simulink model "MLF-VirtualPlatformManualTest"  (R2017b)
settings: Solver=VariableStepAuto  StartTime=0.0  StopTime=inf  RelTol=1e-3
libraries: simulink x3, instrumentlib x2, realtime_pacer_lib x1
settings Model: Creator=twyleg  LastModifiedBy=twyleg

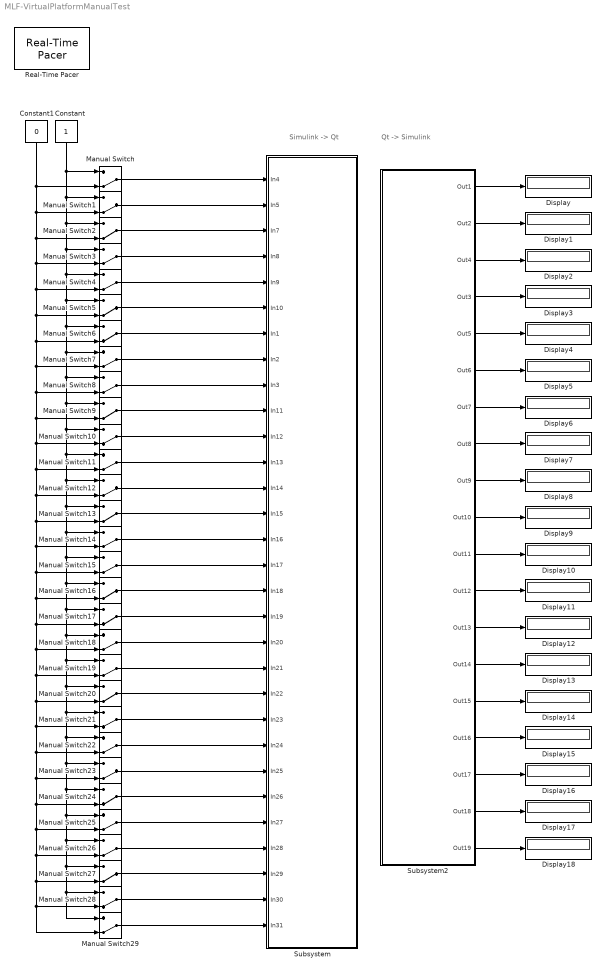
== system MLF-VirtualPlatformManualTest ==
  note: Simulink -> Qt
  note: Qt -> Simulink
  Constant : Constant  OutDataTypeStr=boolean
  Constant1 : Constant  Value=0  OutDataTypeStr=boolean
  Display{,1..18} (19 alike) : Display
  Manual Switch{,1..29} (30 alike) : ManualSwitch  CurrentSetting=0
  Real-Time Pacer : realtime_pacer_lib/Real-Time Pacer  simTimePerRealTime=1
  Subsystem : Subsystem
  Subsystem2 : Subsystem
  wires:
  Subsystem2/1(Out1) -> Display/1
  Subsystem2/2(Out2) -> Display1/1
  Subsystem2/3(Out4) -> Display2/1
  Subsystem2/4(Out3) -> Display3/1
  Subsystem2/5(Out5) -> Display4/1
  Manual Switch/1 -> Subsystem/1(In4)
  Manual Switch1/1 -> Subsystem/2(In5)
  Manual Switch2/1 -> Subsystem/3(In7)
  Manual Switch3/1 -> Subsystem/4(In8)
  Manual Switch4/1 -> Subsystem/5(In9)
  Manual Switch5/1 -> Subsystem/6(In10)
  Manual Switch6/1 -> Subsystem/7(In1)
  Manual Switch7/1 -> Subsystem/8(In2)
  Manual Switch8/1 -> Subsystem/9(In3)
  Manual Switch9/1 -> Subsystem/10(In11)
  Manual Switch10/1 -> Subsystem/11(In12)
  Manual Switch11/1 -> Subsystem/12(In13)
  Manual Switch12/1 -> Subsystem/13(In14)
  Manual Switch13/1 -> Subsystem/14(In15)
  Manual Switch14/1 -> Subsystem/15(In16)
  Manual Switch15/1 -> Subsystem/16(In17)
  Manual Switch16/1 -> Subsystem/17(In18)
  Manual Switch17/1 -> Subsystem/18(In19)
  Manual Switch18/1 -> Subsystem/19(In20)
  Manual Switch19/1 -> Subsystem/20(In21)
  Manual Switch20/1 -> Subsystem/21(In22)
  Manual Switch21/1 -> Subsystem/22(In23)
  Manual Switch22/1 -> Subsystem/23(In24)
  Manual Switch23/1 -> Subsystem/24(In25)
  Manual Switch24/1 -> Subsystem/25(In26)
  Manual Switch25/1 -> Subsystem/26(In27)
  Manual Switch26/1 -> Subsystem/27(In28)
  Manual Switch27/1 -> Subsystem/28(In29)
  Manual Switch28/1 -> Subsystem/29(In30)
  Manual Switch29/1 -> Subsystem/30(In31)
  Constant1/1 -> Manual Switch5/2, Manual Switch6/2, Manual Switch7/2, Manual Switch8/2, Manual Switch9/2, Manual Switch10/2, Manual Switch11/2, Manual Switch12/2, Manual Switch13/2, Manual Switch14/2, Manual Switch15/2, Manual Switch16/2, Manual Switch17/2, Manual Switch18/2, Manual Switch19/2, Manual Switch20/2, Manual Switch21/2, Manual Switch22/2, Manual Switch23/2, Manual Switch24/2, Manual Switch25/2, Manual Switch26/2, Manual Switch27/2, Manual Switch28/2, Manual Switch29/2, Manual Switch4/2, Manual Switch3/2, Manual Switch2/2, Manual Switch1/2, Manual Switch/2
  Constant/1 -> Manual Switch/1, Manual Switch5/1, Manual Switch6/1, Manual Switch7/1, Manual Switch8/1, Manual Switch9/1, Manual Switch10/1, Manual Switch11/1, Manual Switch12/1, Manual Switch13/1, Manual Switch14/1, Manual Switch15/1, Manual Switch16/1, Manual Switch17/1, Manual Switch18/1, Manual Switch19/1, Manual Switch20/1, Manual Switch21/1, Manual Switch22/1, Manual Switch23/1, Manual Switch24/1, Manual Switch25/1, Manual Switch26/1, Manual Switch27/1, Manual Switch28/1, Manual Switch29/1, Manual Switch4/1, Manual Switch3/1, Manual Switch2/1, Manual Switch1/1
  Subsystem2/6(Out6) -> Display5/1
  Subsystem2/7(Out7) -> Display6/1
  Subsystem2/8(Out8) -> Display7/1
  Subsystem2/9(Out9) -> Display8/1
  Subsystem2/10(Out10) -> Display9/1
  Subsystem2/11(Out11) -> Display10/1
  Subsystem2/12(Out12) -> Display11/1
  Subsystem2/13(Out13) -> Display12/1
  Subsystem2/14(Out14) -> Display13/1
  Subsystem2/15(Out15) -> Display14/1
  Subsystem2/16(Out16) -> Display15/1
  Subsystem2/17(Out17) -> Display16/1
  Subsystem2/18(Out18) -> Display17/1
  Subsystem2/19(Out19) -> Display18/1

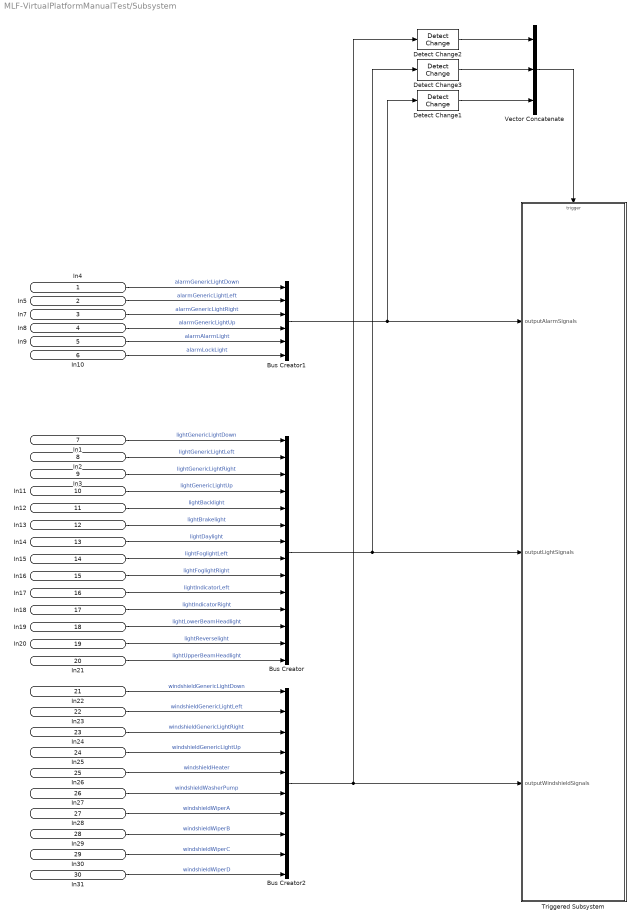
== system MLF-VirtualPlatformManualTest/Subsystem ==
  In4 : Inport
  In5 : Inport  Port=2
  In7 : Inport  Port=3
  In8 : Inport  Port=4
  In9 : Inport  Port=5
  In10 : Inport  Port=6
  In1 : Inport  Port=7
  In2 : Inport  Port=8
  In3 : Inport  Port=9
  In11 : Inport  Port=10
  In12 : Inport  Port=11
  In13 : Inport  Port=12
  In14 : Inport  Port=13
  In15 : Inport  Port=14
  In16 : Inport  Port=15
  In17 : Inport  Port=16
  In18 : Inport  Port=17
  In19 : Inport  Port=18
  In20 : Inport  Port=19
  In21 : Inport  Port=20
  In22 : Inport  Port=21
  In23 : Inport  Port=22
  In24 : Inport  Port=23
  In25 : Inport  Port=24
  In26 : Inport  Port=25
  In27 : Inport  Port=26
  In28 : Inport  Port=27
  In29 : Inport  Port=28
  In30 : Inport  Port=29
  In31 : Inport  Port=30
  Bus Creator : BusCreator  Inputs=14
  Bus Creator1 : BusCreator  Inputs=6
  Bus Creator2 : BusCreator  Inputs=10
  Detect Change1 : simulink/Logic and Bit Operations/Detect Change  vinit=0  OutDataTypeStr=boolean
  Detect Change2 : simulink/Logic and Bit Operations/Detect Change  vinit=0  OutDataTypeStr=boolean
  Detect Change3 : simulink/Logic and Bit Operations/Detect Change  vinit=0  OutDataTypeStr=boolean
  Triggered Subsystem : Subsystem  TreatAsAtomicUnit=on
  Vector Concatenate : Concatenate  NumInputs=3
  wires:
  Bus Creator/1 -> Detect Change3/1, Triggered Subsystem/2("outputLightSignals ")
  In1/1 -> Bus Creator/1  "lightGenericLightDown"
  In2/1 -> Bus Creator/2  "lightGenericLightLeft"
  In3/1 -> Bus Creator/3  "lightGenericLightRight"
  Detect Change3/1 -> Vector Concatenate/2
  In4/1 -> Bus Creator1/1  "alarmGenericLightDown"
  In5/1 -> Bus Creator1/2  "alarmGenericLightLeft"
  Bus Creator1/1 -> Detect Change1/1, Triggered Subsystem/1(outputAlarmSignals)
  Detect Change1/1 -> Vector Concatenate/3
  Vector Concatenate/1 -> Triggered Subsystem/Trigger
  In7/1 -> Bus Creator1/3  "alarmGenericLightRight"
  In8/1 -> Bus Creator1/4  "alarmGenericLightUp"
  In9/1 -> Bus Creator1/5  "alarmAlarmLight"
  In10/1 -> Bus Creator1/6  "alarmLockLight"
  Bus Creator2/1 -> Detect Change2/1, Triggered Subsystem/3(outputWindshieldSignals)
  Detect Change2/1 -> Vector Concatenate/1
  In11/1 -> Bus Creator/4  "lightGenericLightUp"
  In12/1 -> Bus Creator/5  "lightBacklight"
  In13/1 -> Bus Creator/6  "lightBrakelight"
  In14/1 -> Bus Creator/7  "lightDaylight"
  In15/1 -> Bus Creator/8  "lightFoglightLeft"
  In16/1 -> Bus Creator/9  "lightFoglightRight"
  In17/1 -> Bus Creator/10  "lightIndicatorLeft"
  In18/1 -> Bus Creator/11  "lightIndicatorRight"
  In19/1 -> Bus Creator/12  "lightLowerBeamHeadlight"
  In21/1 -> Bus Creator/14  "lightUpperBeamHeadlight"
  In20/1 -> Bus Creator/13  "lightReverselight"
  In22/1 -> Bus Creator2/1  "windshieldGenericLightDown"
  In23/1 -> Bus Creator2/2  "windshieldGenericLightLeft"
  In24/1 -> Bus Creator2/3  "windshieldGenericLightRight"
  In25/1 -> Bus Creator2/4  "windshieldGenericLightUp"
  In26/1 -> Bus Creator2/5  "windshieldHeater"
  In27/1 -> Bus Creator2/6  "windshieldWasherPump"
  In28/1 -> Bus Creator2/7  "windshieldWiperA"
  In29/1 -> Bus Creator2/8  "windshieldWiperB"
  In30/1 -> Bus Creator2/9  "windshieldWiperC"
  In31/1 -> Bus Creator2/10  "windshieldWiperD"

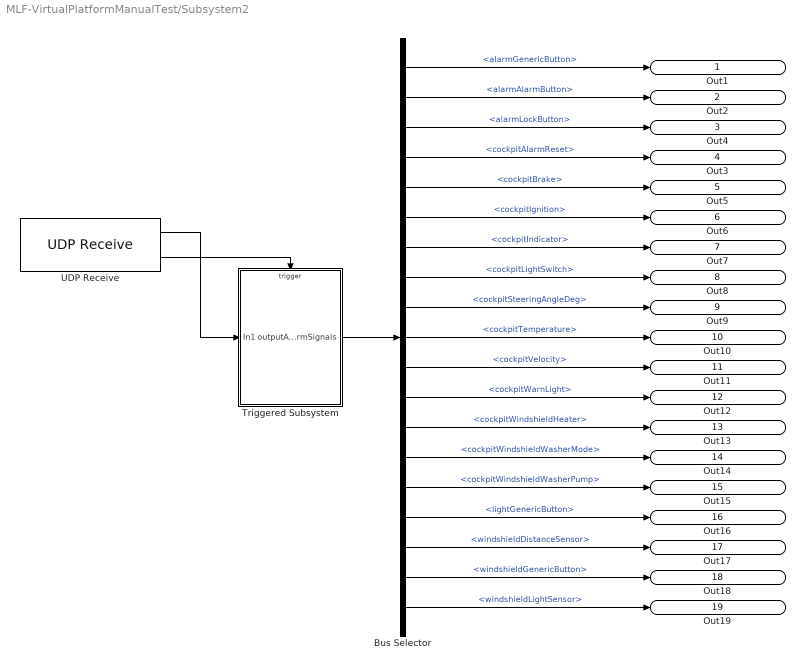
== system MLF-VirtualPlatformManualTest/Subsystem2 ==
  Bus Selector : BusSelector  OutputSignals=alarmGenericButton,alarmAlarmButton,alarmLockButton,cockpitAlarmReset,cockpitBrake,cockpitIgnition,cockpitIndicator,cockpitLightSwitch,cockpitSteeringAngleDeg,cockpitTemperature,cockpitVelocity,cockpitWarnLight,cockpitWindshieldHeater,cockpitWindshieldWasherMode,cockpitWindshieldWasherPump,lightGenericButton,windshieldDistanceSensor,windshieldGenericButton,windshieldLightSensor
  Triggered Subsystem : Subsystem  TreatAsAtomicUnit=on
  UDP Receive : instrumentlib/UDP Receive  Host=10.0.2.2  Port=50001  LocalPort=50001  DataSize=4096  EnableBlockingMode=off  Timeout=10  SampleTime=0.01  DataType=uint8  ByteOrder=BigEndian
      settings: SourceProductName=Instrument Control Toolbox
  Out1 : Outport
  Out2 : Outport  Port=2
  Out4 : Outport  Port=3
  Out3 : Outport  Port=4
  Out5 : Outport  Port=5
  Out6 : Outport  Port=6
  Out7 : Outport  Port=7
  Out8 : Outport  Port=8
  Out9 : Outport  Port=9
  Out10 : Outport  Port=10
  Out11 : Outport  Port=11
  Out12 : Outport  Port=12
  Out13 : Outport  Port=13
  Out14 : Outport  Port=14
  Out15 : Outport  Port=15
  Out16 : Outport  Port=16
  Out17 : Outport  Port=17
  Out18 : Outport  Port=18
  Out19 : Outport  Port=19
  wires:
  UDP Receive/2 -> Triggered Subsystem/Trigger
  UDP Receive/1 -> Triggered Subsystem/1(In1)
  Triggered Subsystem/1(outputAlarmSignals) -> Bus Selector/1
  Bus Selector/1 -> Out1/1  "<alarmGenericButton>"
  Bus Selector/2 -> Out2/1  "<alarmAlarmButton>"
  Bus Selector/3 -> Out4/1  "<alarmLockButton>"
  Bus Selector/4 -> Out3/1  "<cockpitAlarmReset>"
  Bus Selector/5 -> Out5/1  "<cockpitBrake>"
  Bus Selector/6 -> Out6/1  "<cockpitIgnition>"
  Bus Selector/7 -> Out7/1  "<cockpitIndicator>"
  Bus Selector/19 -> Out19/1  "<windshieldLightSensor>"
  Bus Selector/18 -> Out18/1  "<windshieldGenericButton>"
  Bus Selector/17 -> Out17/1  "<windshieldDistanceSensor>"
  Bus Selector/16 -> Out16/1  "<lightGenericButton>"
  Bus Selector/15 -> Out15/1  "<cockpitWindshieldWasherPump>"
  Bus Selector/14 -> Out14/1  "<cockpitWindshieldWasherMode>"
  Bus Selector/13 -> Out13/1  "<cockpitWindshieldHeater>"
  Bus Selector/12 -> Out12/1  "<cockpitWarnLight>"
  Bus Selector/11 -> Out11/1  "<cockpitVelocity>"
  Bus Selector/10 -> Out10/1  "<cockpitTemperature>"
  Bus Selector/9 -> Out9/1  "<cockpitSteeringAngleDeg>"
  Bus Selector/8 -> Out8/1  "<cockpitLightSwitch>"

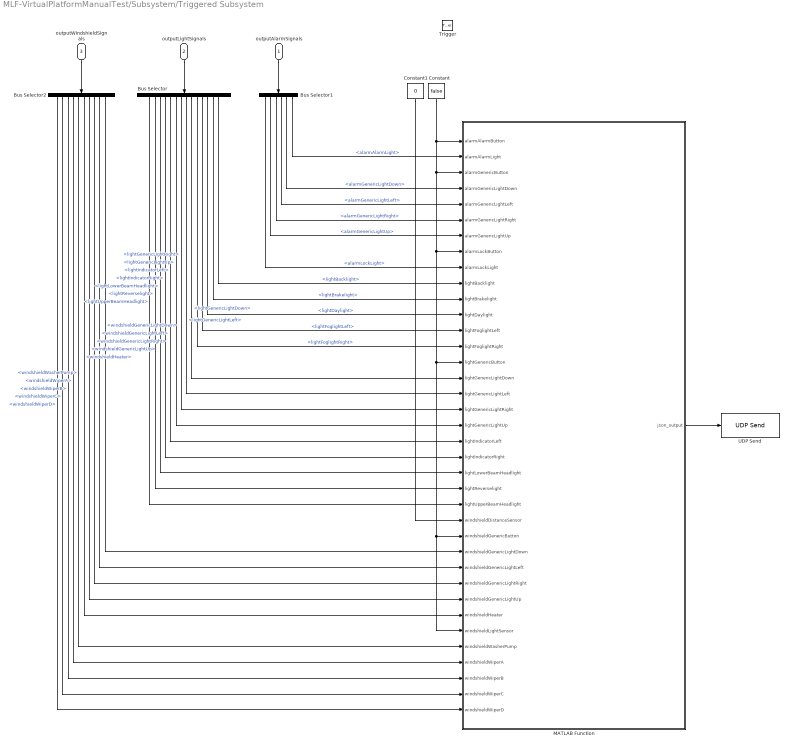
== system MLF-VirtualPlatformManualTest/Subsystem/Triggered Subsystem ==
  outputAlarmSignals : Inport
  "outputLightSignals " : Inport  Port=2  OutDataTypeStr=boolean
  outputWindshieldSignals : Inport  Port=3  OutDataTypeStr=boolean
  Trigger : TriggerPort  VariantControl=Variant
  Bus Selector : BusSelector  OutputSignals=lightUpperBeamHeadlight,lightReverselight,lightLowerBeamHeadlight,lightIndicatorRight,lightIndicatorLeft,lightGenericLightUp,lightGenericLightRight,lightGenericLightLeft,lightGenericLightDown,lightFoglightRight,lightFoglightLeft,lightDaylight,lightBrakelight,lightBacklight
  Bus Selector1 : BusSelector  OutputSignals=alarmLockLight,alarmGenericLightUp,alarmGenericLightRight,alarmGenericLightLeft,alarmGenericLightDown,alarmAlarmLight
  Bus Selector2 : BusSelector  OutputSignals=windshieldWiperD,windshieldWiperC,windshieldWiperB,windshieldWiperA,windshieldWasherPump,windshieldHeater,windshieldGenericLightUp,windshieldGenericLightRight,windshieldGenericLightLeft,windshieldGenericLightDown
  Constant : Constant  Value=false  OutDataTypeStr=boolean
  Constant1 : Constant  Value=0
  MATLAB Function : MATLAB Function  TreatAsAtomicUnit=on
  UDP Send : instrumentlib/UDP Send  Host=192.168.1.121  Port=50000  LocalPort=-1  EnableBlockingMode=on  ByteOrder=BigEndian
      settings: SourceProductName=Instrument Control Toolbox
  wires:
  MATLAB Function/1(json_output) -> UDP Send/1
  "outputLightSignals "/1 -> Bus Selector/1
  outputAlarmSignals/1 -> Bus Selector1/1
  Constant/1 -> MATLAB Function/1(alarmAlarmButton), MATLAB Function/3(alarmGenericButton), MATLAB Function/8(alarmLockButton), MATLAB Function/32(windshieldLightSensor), MATLAB Function/26(windshieldGenericButton), MATLAB Function/15(lightGenericButton)
  Constant1/1 -> MATLAB Function/25(windshieldDistanceSensor)
  Bus Selector1/6 -> MATLAB Function/2(alarmAlarmLight)  "<alarmAlarmLight>"
  Bus Selector1/5 -> MATLAB Function/4(alarmGenericLightDown)  "<alarmGenericLightDown>"
  Bus Selector1/4 -> MATLAB Function/5(alarmGenericLightLeft)  "<alarmGenericLightLeft>"
  Bus Selector1/3 -> MATLAB Function/6(alarmGenericLightRight)  "<alarmGenericLightRight>"
  Bus Selector1/2 -> MATLAB Function/7(alarmGenericLightUp)  "<alarmGenericLightUp>"
  Bus Selector1/1 -> MATLAB Function/9(alarmLockLight)  "<alarmLockLight>"
  Bus Selector/14 -> MATLAB Function/10(lightBacklight)  "<lightBacklight>"
  Bus Selector/13 -> MATLAB Function/11(lightBrakelight)  "<lightBrakelight>"
  Bus Selector/12 -> MATLAB Function/12(lightDaylight)  "<lightDaylight>"
  Bus Selector/11 -> MATLAB Function/13(lightFoglightLeft)  "<lightFoglightLeft>"
  Bus Selector/9 -> MATLAB Function/16(lightGenericLightDown)  "<lightGenericLightDown>"
  Bus Selector/10 -> MATLAB Function/14(lightFoglightRight)  "<lightFoglightRight>"
  Bus Selector/8 -> MATLAB Function/17(lightGenericLightLeft)  "<lightGenericLightLeft>"
  Bus Selector/7 -> MATLAB Function/18(lightGenericLightRight)  "<lightGenericLightRight>"
  Bus Selector/6 -> MATLAB Function/19(lightGenericLightUp)  "<lightGenericLightUp>"
  Bus Selector/5 -> MATLAB Function/20(lightIndicatorLeft)  "<lightIndicatorLeft>"
  Bus Selector/4 -> MATLAB Function/21(lightIndicatorRight)  "<lightIndicatorRight>"
  Bus Selector/3 -> MATLAB Function/22(lightLowerBeamHeadlight)  "<lightLowerBeamHeadlight>"
  Bus Selector/2 -> MATLAB Function/23(lightReverselight)  "<lightReverselight>"
  Bus Selector/1 -> MATLAB Function/24(lightUpperBeamHeadlight)  "<lightUpperBeamHeadlight>"
  outputWindshieldSignals/1 -> Bus Selector2/1
  Bus Selector2/10 -> MATLAB Function/27(windshieldGenericLightDown)  "<windshieldGenericLightDown>"
  Bus Selector2/9 -> MATLAB Function/28(windshieldGenericLightLeft)  "<windshieldGenericLightLeft>"
  Bus Selector2/8 -> MATLAB Function/29(windshieldGenericLightRight)  "<windshieldGenericLightRight>"
  Bus Selector2/7 -> MATLAB Function/30(windshieldGenericLightUp)  "<windshieldGenericLightUp>"
  Bus Selector2/6 -> MATLAB Function/31(windshieldHeater)  "<windshieldHeater>"
  Bus Selector2/5 -> MATLAB Function/33(windshieldWasherPump)  "<windshieldWasherPump>"
  Bus Selector2/4 -> MATLAB Function/34(windshieldWiperA)  "<windshieldWiperA>"
  Bus Selector2/3 -> MATLAB Function/35(windshieldWiperB)  "<windshieldWiperB>"
  Bus Selector2/2 -> MATLAB Function/36(windshieldWiperC)  "<windshieldWiperC>"
  Bus Selector2/1 -> MATLAB Function/37(windshieldWiperD)  "<windshieldWiperD>"

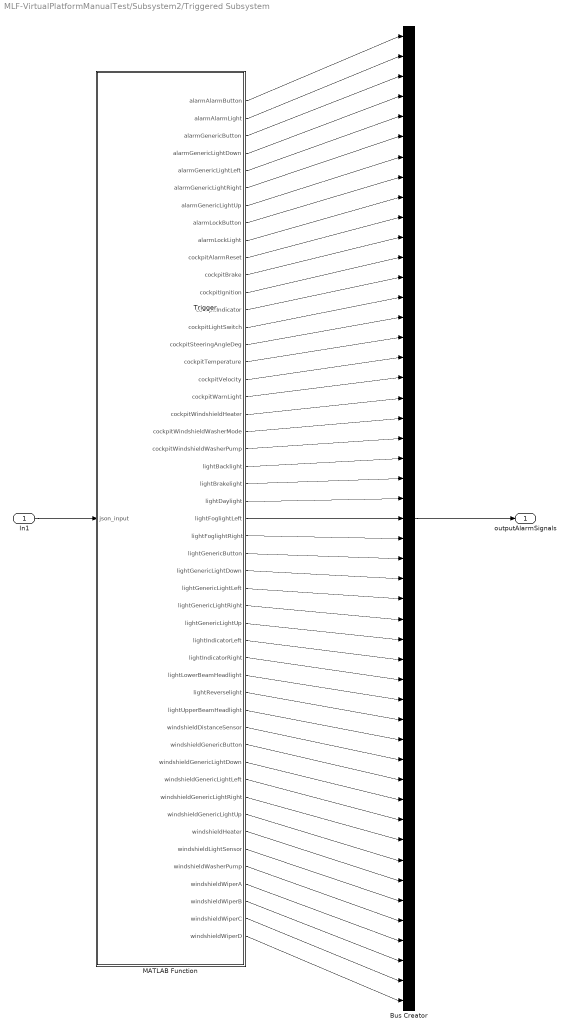
== system MLF-VirtualPlatformManualTest/Subsystem2/Triggered Subsystem ==
  In1 : Inport
  Trigger : TriggerPort  VariantControl=Variant
  Bus Creator : BusCreator  Inputs=49
  MATLAB Function : MATLAB Function  TreatAsAtomicUnit=on
  outputAlarmSignals : Outport
  wires:
  In1/1 -> MATLAB Function/1(json_input)
  Bus Creator/1 -> outputAlarmSignals/1
  MATLAB Function/1(alarmAlarmButton) -> Bus Creator/1
  MATLAB Function/2(alarmAlarmLight) -> Bus Creator/2
  MATLAB Function/3(alarmGenericButton) -> Bus Creator/3
  MATLAB Function/4(alarmGenericLightDown) -> Bus Creator/4
  MATLAB Function/5(alarmGenericLightLeft) -> Bus Creator/5
  MATLAB Function/6(alarmGenericLightRight) -> Bus Creator/6
  MATLAB Function/7(alarmGenericLightUp) -> Bus Creator/7
  MATLAB Function/8(alarmLockButton) -> Bus Creator/8
  MATLAB Function/9(alarmLockLight) -> Bus Creator/9
  MATLAB Function/10(cockpitAlarmReset) -> Bus Creator/10
  MATLAB Function/11(cockpitBrake) -> Bus Creator/11
  MATLAB Function/13(cockpitIndicator) -> Bus Creator/13
  MATLAB Function/12(cockpitIgnition) -> Bus Creator/12
  MATLAB Function/14(cockpitLightSwitch) -> Bus Creator/14
  MATLAB Function/15(cockpitSteeringAngleDeg) -> Bus Creator/15
  MATLAB Function/16(cockpitTemperature) -> Bus Creator/16
  MATLAB Function/17(cockpitVelocity) -> Bus Creator/17
  MATLAB Function/18(cockpitWarnLight) -> Bus Creator/18
  MATLAB Function/19(cockpitWindshieldHeater) -> Bus Creator/19
  MATLAB Function/20(cockpitWindshieldWasherMode) -> Bus Creator/20
  MATLAB Function/21(cockpitWindshieldWasherPump) -> Bus Creator/21
  MATLAB Function/22(lightBacklight) -> Bus Creator/22
  MATLAB Function/23(lightBrakelight) -> Bus Creator/23
  MATLAB Function/24(lightDaylight) -> Bus Creator/24
  MATLAB Function/25(lightFoglightLeft) -> Bus Creator/25
  MATLAB Function/26(lightFoglightRight) -> Bus Creator/26
  MATLAB Function/27(lightGenericButton) -> Bus Creator/27
  MATLAB Function/29(lightGenericLightLeft) -> Bus Creator/29
  MATLAB Function/28(lightGenericLightDown) -> Bus Creator/28
  MATLAB Function/30(lightGenericLightRight) -> Bus Creator/30
  MATLAB Function/31(lightGenericLightUp) -> Bus Creator/31
  MATLAB Function/32(lightIndicatorLeft) -> Bus Creator/32
  MATLAB Function/33(lightIndicatorRight) -> Bus Creator/33
  MATLAB Function/34(lightLowerBeamHeadlight) -> Bus Creator/34
  MATLAB Function/35(lightReverselight) -> Bus Creator/35
  MATLAB Function/36(lightUpperBeamHeadlight) -> Bus Creator/36
  MATLAB Function/37(windshieldDistanceSensor) -> Bus Creator/37
  MATLAB Function/38(windshieldGenericButton) -> Bus Creator/38
  MATLAB Function/39(windshieldGenericLightDown) -> Bus Creator/39
  MATLAB Function/40(windshieldGenericLightLeft) -> Bus Creator/40
  MATLAB Function/41(windshieldGenericLightRight) -> Bus Creator/41
  MATLAB Function/42(windshieldGenericLightUp) -> Bus Creator/42
  MATLAB Function/43(windshieldHeater) -> Bus Creator/43
  MATLAB Function/44(windshieldLightSensor) -> Bus Creator/44
  MATLAB Function/45(windshieldWasherPump) -> Bus Creator/45
  MATLAB Function/46(windshieldWiperA) -> Bus Creator/46
  MATLAB Function/47(windshieldWiperB) -> Bus Creator/47
  MATLAB Function/48(windshieldWiperC) -> Bus Creator/48
  MATLAB Function/49(windshieldWiperD) -> Bus Creator/49

== matlab function MLF-VirtualPlatformManualTest/Subsystem/Triggered Subsystem/MATLAB Function ==
  data: alarmAlarmButton input; alarmAlarmLight input; alarmGenericButton input; alarmGenericLightDown input; alarmGenericLightLeft input; alarmGenericLightRight input; alarmGenericLightUp input; alarmLockButton input; alarmLockLight input; lightBacklight input; lightBrakelight input; lightDaylight input; json_output output size=4096; lightFoglightLeft input; lightFoglightRight input; lightGenericButton input; lightGenericLightDown input; lightGenericLightLeft input; lightGenericLightRight input; lightGenericLightUp input; lightIndicatorLeft input; lightIndicatorRight input; lightLowerBeamHeadlight input; lightReverselight input; lightUpperBeamHeadlight input; windshieldDistanceSensor input; windshieldGenericButton input; windshieldGenericLightDown input; windshieldGenericLightLeft input; windshieldGenericLightRight input; windshieldGenericLightUp input; windshieldHeater input; windshieldLightSensor input; windshieldWasherPump input; windshieldWiperA input; windshieldWiperB input; windshieldWiperC input; windshieldWiperD input
function json_output = fcn( ...
    alarmAlarmButton, ...
    alarmAlarmLight, ...
    alarmGenericButton, ...
    alarmGenericLightDown, ...
    alarmGenericLightLeft, ...
    alarmGenericLightRight, ...
    alarmGenericLightUp, ...
    alarmLockButton, ...
    alarmLockLight, ...
    lightBacklight, ...
    lightBrakelight, ...
    lightDaylight, ...
    lightFoglightLeft, ...
    lightFoglightRight, ...
    lightGenericButton, ...
    lightGenericLightDown, ...
    lightGenericLightLeft, ...
    lightGenericLightRight, ...
    lightGenericLightUp, ...
    lightIndicatorLeft, ...
    lightIndicatorRight, ...
    lightLowerBeamHeadlight, ...
    lightReverselight, ...
    lightUpperBeamHeadlight, ...
    windshieldDistanceSensor, ...
    windshieldGenericButton, ...
    windshieldGenericLightDown, ...
    windshieldGenericLightLeft, ...
    windshieldGenericLightRight, ...
    windshieldGenericLightUp, ...
    windshieldHeater, ...
    windshieldLightSensor, ...
    windshieldWasherPump, ...
    windshieldWiperA, ...
    windshieldWiperB, ...
    windshieldWiperC, ...
    windshieldWiperD)

coder.extrinsic('jsonencode')

% Allocate output array size an initialize with zeroes
json_output = zeros(4096,1,'uint8');


% Prepare the data
json_struct = struct(...
    'alarmAlarmButton', alarmAlarmButton, ...
    'alarmAlarmLight', alarmAlarmLight, ...
    'alarmGenericButton', alarmGenericButton, ...
    'alarmGenericLightDown', alarmGenericLightDown, ...
    'alarmGenericLightLeft', alarmGenericLightLeft, ...
    'alarmGenericLightRight', alarmGenericLightRight, ...
    'alarmGenericLightUp', alarmGenericLightUp, ...
    'alarmLockButton', alarmLockButton, ...
    'alarmLockLight', alarmLockLight, ...
    'lightBacklight',lightBacklight, ...
    'lightBrakelight',lightBrakelight, ...
    'lightDaylight',lightDaylight, ...
    'lightFoglightLeft', lightFoglightLeft, ...
    'lightFoglightRight', lightFoglightRight, ...
    'lightGenericButton', lightGenericButton, ...
    'lightGenericLightDown', lightGenericLightDown, ...
    'lightGenericLightLeft', lightGenericLightLeft, ...
    'lightGenericLightRight', lightGenericLightRight, ...
    'lightGenericLightUp', lightGenericLightUp, ...
    'lightIndicatorLeft', lightIndicatorLeft, ...
    'lightIndicatorRight', lightIndicatorRight, ...
    'lightLowerBeamHeadlight', lightLowerBeamHeadlight, ...
    'lightReverselight', lightReverselight, ...
    'lightUpperBeamHeadlight', lightUpperBeamHeadlight, ...
    'windshieldDistanceSensor', windshieldDistanceSensor, ...
    'windshieldGenericButton', windshieldGenericButton, ...
    'windshieldGenericLightDown', windshieldGenericLightDown, ...
    'windshieldGenericLightLeft', windshieldGenericLightLeft, ...
    'windshieldGenericLightRight', windshieldGenericLightRight, ...
    'windshieldGenericLightUp', windshieldGenericLightUp, ...
    'windshieldHeater', windshieldHeater, ...
    'windshieldLightSensor', windshieldLightSensor, ...
    'windshieldWasherPump', windshieldWasherPump, ...
    'windshieldWiperA', windshieldWiperA, ...
    'windshieldWiperB', windshieldWiperB, ...
    'windshieldWiperC', windshieldWiperC, ...
    'windshieldWiperD', windshieldWiperD ...
)

% Create json string from data
json_string = jsonencode(json_struct)

% Get length of final json string
len = uint16(0)
len = uint16(length(json_string))

% Copy json string char by char to output string
for i = 1:len
    json_output(i) = uint8(json_string(i));
end

json_output(len+1) = uint8(10)

== matlab function MLF-VirtualPlatformManualTest/Subsystem2/Triggered Subsystem/MATLAB Function ==
  data: json_input input; alarmAlarmButton output; alarmAlarmLight output; alarmGenericButton output; alarmGenericLightDown output; alarmGenericLightLeft output; alarmGenericLightRight output; alarmGenericLightUp output; alarmLockButton output; alarmLockLight output; cockpitAlarmReset output; cockpitBrake output; cockpitIgnition output; cockpitIndicator output; cockpitLightSwitch output; cockpitSteeringAngleDeg output; cockpitTemperature output; cockpitVelocity output; cockpitWarnLight output; cockpitWindshieldHeater output; cockpitWindshieldWasherMode output; cockpitWindshieldWasherPump output; lightBacklight output; lightBrakelight output; lightDaylight output; lightFoglightLeft output; lightFoglightRight output; lightGenericButton output; lightGenericLightDown output; lightGenericLightLeft output; lightGenericLightRight output; lightGenericLightUp output; lightIndicatorLeft output; lightIndicatorRight output; lightLowerBeamHeadlight output; lightReverselight output; lightUpperBeamHeadlight output; windshieldDistanceSensor output; windshieldGenericButton output; windshieldGenericLightDown output; windshieldGenericLightLeft output; windshieldGenericLightRight output; windshieldGenericLightUp output; windshieldHeater output; windshieldLightSensor output; windshieldWasherPump output; windshieldWiperA output; windshieldWiperB output; windshieldWiperC output; windshieldWiperD output
function [ ...
    alarmAlarmButton, ...
    alarmAlarmLight, ...
    alarmGenericButton, ...
    alarmGenericLightDown, ...
    alarmGenericLightLeft, ...
    alarmGenericLightRight, ...
    alarmGenericLightUp, ...
    alarmLockButton, ...
    alarmLockLight, ...
    cockpitAlarmReset, ...
    cockpitBrake, ...
    cockpitIgnition, ...
    cockpitIndicator, ...
    cockpitLightSwitch, ...
    cockpitSteeringAngleDeg, ...
    cockpitTemperature, ...
    cockpitVelocity, ...
    cockpitWarnLight, ...
    cockpitWindshieldHeater, ...
    cockpitWindshieldWasherMode, ...
    cockpitWindshieldWasherPump, ...
    lightBacklight, ...
    lightBrakelight, ...
    lightDaylight, ...
    lightFoglightLeft, ...
    lightFoglightRight, ...
    lightGenericButton, ...
    lightGenericLightDown, ...
    lightGenericLightLeft, ...
    lightGenericLightRight, ...
    lightGenericLightUp, ...
    lightIndicatorLeft, ...
    lightIndicatorRight, ...
    lightLowerBeamHeadlight, ...
    lightReverselight, ...
    lightUpperBeamHeadlight, ...
    windshieldDistanceSensor, ...
    windshieldGenericButton, ...
    windshieldGenericLightDown, ...
    windshieldGenericLightLeft, ...
    windshieldGenericLightRight, ...
    windshieldGenericLightUp, ...
    windshieldHeater, ...
    windshieldLightSensor, ...
    windshieldWasherPump, ...
    windshieldWiperA, ...
    windshieldWiperB, ...
    windshieldWiperC, ...
    windshieldWiperD ...
    ] = fcn(json_input)

coder.extrinsic('jsondecode');

%bar = '{"alarmAlarmButton": false,"lightBacklight": true,"lightBrakelight": true,"lightDaylight": true}    '

jsonLen = 0;

for i = 1:length(json_input)
   c = json_input(i);
   if c == 0
        break
   else
        jsonLen = i;
   end
   
end

chr = blanks(jsonLen);

for i = 1:jsonLen
    chr(i) = json_input(i);
end

jsonStruct.alarmAlarmButton = false;
jsonStruct.alarmAlarmLight = false;
jsonStruct.alarmGenericButton = false;
jsonStruct.alarmGenericLightDown = false;
jsonStruct.alarmGenericLightLeft = false;
jsonStruct.alarmGenericLightRight = false;
jsonStruct.alarmGenericLightUp = false;
jsonStruct.alarmLockButton = false;
jsonStruct.alarmLockLight = false;
jsonStruct.cockpitAlarmReset = double(0);
jsonStruct.cockpitBrake = double(0);
jsonStruct.cockpitIgnition = double(0);
jsonStruct.cockpitIndicator = double(0);
jsonStruct.cockpitLightSwitch = double(0);
jsonStruct.cockpitSteeringAngleDeg = double(0);
jsonStruct.cockpitTemperature = double(0);
jsonStruct.cockpitVelocity = double(0);
jsonStruct.cockpitWarnLight = double(0);
jsonStruct.cockpitWindshieldHeater = double(0);
jsonStruct.cockpitWindshieldWasherMode = double(0);
jsonStruct.cockpitWindshieldWasherPump = double(0);
jsonStruct.lightBacklight = false;
jsonStruct.lightBrakelight = false;
jsonStruct.lightDaylight = false;
jsonStruct.lightFoglightLeft = false;
jsonStruct.lightFoglightRight = false;
jsonStruct.lightGenericButton = false;
jsonStruct.lightGenericLightDown = false;
jsonStruct.lightGenericLightLeft = false;
jsonStruct.lightGenericLightRight = false;
jsonStruct.lightGenericLightUp = false;
jsonStruct.lightIndicatorLeft = false;
jsonStruct.lightIndicatorRight = false;
jsonStruct.lightLowerBeamHeadlight = false;
jsonStruct.lightReverselight = false;
jsonStruct.lightUpperBeamHeadlight = false;
jsonStruct.windshieldDistanceSensor = double(0);
jsonStruct.windshieldGenericButton = false;
jsonStruct.windshieldGenericLightDown = false;
jsonStruct.windshieldGenericLightLeft = false;
jsonStruct.windshieldGenericLightRight = false;
jsonStruct.windshieldGenericLightUp = false;
jsonStruct.windshieldHeater = false;
jsonStruct.windshieldLightSensor = false;
jsonStruct.windshieldWasherPump = false;
jsonStruct.windshieldWiperA = false;
jsonStruct.windshieldWiperB = false;
jsonStruct.windshieldWiperC = false;
jsonStruct.windshieldWiperD = false;

jsonStruct = jsondecode(chr);

alarmAlarmButton = jsonStruct.alarmAlarmButton;
alarmAlarmLight = jsonStruct.alarmAlarmLight;
alarmGenericButton = jsonStruct.alarmGenericButton;
alarmGenericLightDown = jsonStruct.alarmGenericLightDown;
alarmGenericLightLeft = jsonStruct.alarmGenericLightLeft;
alarmGenericLightRight = jsonStruct.alarmGenericLightRight;
alarmGenericLightUp = jsonStruct.alarmGenericLightUp;
alarmLockButton = jsonStruct.alarmLockButton;
alarmLockLight = jsonStruct.alarmLockLight;
cockpitAlarmReset = jsonStruct.cockpitAlarmReset;
cockpitBrake = jsonStruct.cockpitBrake;
cockpitIgnition = jsonStruct.cockpitIgnition;
cockpitIndicator = jsonStruct.cockpitIndicator;
cockpitLightSwitch = jsonStruct.cockpitLightSwitch;
cockpitSteeringAngleDeg = jsonStruct.cockpitSteeringAngleDeg;
cockpitTemperature = jsonStruct.cockpitTemperature;
cockpitVelocity = jsonStruct.cockpitVelocity;
cockpitWarnLight = jsonStruct.cockpitWarnLight;
cockpitWindshieldHeater = jsonStruct.cockpitWindshieldHeater;
cockpitWindshieldWasherMode = jsonStruct.cockpitWindshieldWasherMode;
cockpitWindshieldWasherPump = jsonStruct.cockpitWindshieldWasherPump;
lightBacklight = jsonStruct.lightBacklight;
lightBrakelight = jsonStruct.lightBrakelight;
lightDaylight = jsonStruct.lightDaylight;
lightFoglightLeft = jsonStruct.lightFoglightLeft;
lightFoglightRight = jsonStruct.lightFoglightRight;
lightGenericButton = jsonStruct.lightGenericButton;
lightGenericLightDown = jsonStruct.lightGenericLightDown;
lightGenericLightLeft = jsonStruct.lightGenericLightLeft;
lightGenericLightRight = jsonStruct.lightGenericLightRight;
lightGenericLightUp = jsonStruct.lightGenericLightUp;
lightIndicatorLeft = jsonStruct.lightIndicatorLeft;
lightIndicatorRight = jsonStruct.lightIndicatorRight;
lightLowerBeamHeadlight = jsonStruct.lightLowerBeamHeadlight;
lightReverselight = jsonStruct.lightReverselight;
lightUpperBeamHeadlight = jsonStruct.lightUpperBeamHeadlight;
windshieldDistanceSensor = jsonStruct.windshieldDistanceSensor;
windshieldGenericButton = jsonStruct.windshieldGenericButton;
windshieldGenericLightDown = jsonStruct.windshieldGenericLightDown;
windshieldGenericLightLeft = jsonStruct.windshieldGenericLightLeft;
windshieldGenericLightRight = jsonStruct.windshieldGenericLightRight;
windshieldGenericLightUp = jsonStruct.windshieldGenericLightUp;
windshieldHeater = jsonStruct.windshieldHeater;
windshieldLightSensor = jsonStruct.windshieldLightSensor;
windshieldWasherPump = jsonStruct.windshieldWasherPump;
windshieldWiperA = jsonStruct.windshieldWiperA;
windshieldWiperB = jsonStruct.windshieldWiperB;
windshieldWiperC = jsonStruct.windshieldWiperC;
windshieldWiperD = jsonStruct.windshieldWiperD;
